simulink model "Bernabe_Simulink3"  (R2023b)
settings: Solver=VariableStepAuto  StartTime=0.0  StopTime=20  RelTol=1e-3
values from neighbouring files (symbols this model uses):
  G_den3 = [1 2 1]    [Bernabe_No.3&4.m]
  G_num3 = [1]    [Bernabe_No.3&4.m]
settings Model: Creator=Abegale Bernabe  LastModifiedBy=Abegale Bernabe

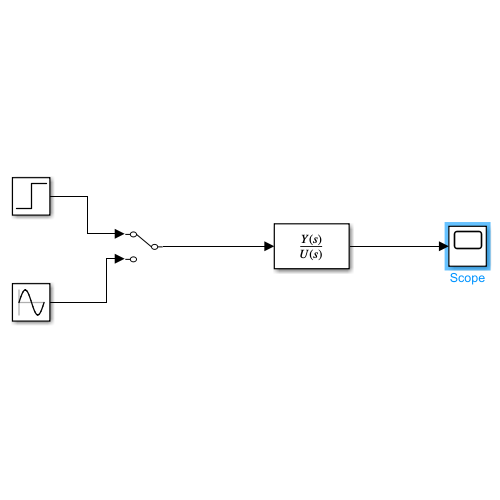
[thumbnail: Simulink's stored preview of the top-level diagram]
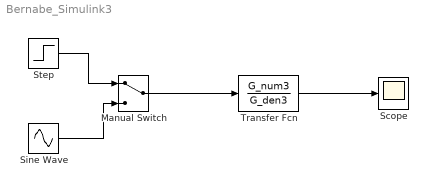
== system Bernabe_Simulink3 ==
  Manual Switch : ManualSwitch
  Scope : Scope
  Sine Wave : Sin  SampleTime=0
  Step : Step  Time=0  SampleTime=0
  Transfer Fcn : TransferFcn  Numerator=G_num3  Denominator=G_den3
  wires:
  Step/1 -> Manual Switch/1
  Sine Wave/1 -> Manual Switch/2
  Manual Switch/1 -> Transfer Fcn/1
  Transfer Fcn/1 -> Scope/1
